simulink model "path_following_PID_v2"  (R2021b)
settings: Solver=VariableStepAuto  StartTime=0.0  StopTime=4000  RelTol=1e-3
model workspace (MAT data in the model file):
  index = 1
values from neighbouring files (symbols this model uses):
  ref = [x_ref, -y_ref]    [reference.m]
libraries: slpidlib x2
settings Model: Creator=andreagottardini  LastModifiedBy=Utente
settings DataIOCC: ReturnWorkspaceOutputs=off
settings DebuggingCC: UnconnectedInputMsg=none  UnconnectedOutputMsg=none  UnconnectedLineMsg=none
settings RTWCC: DLArmComputeVersion=20.02.1

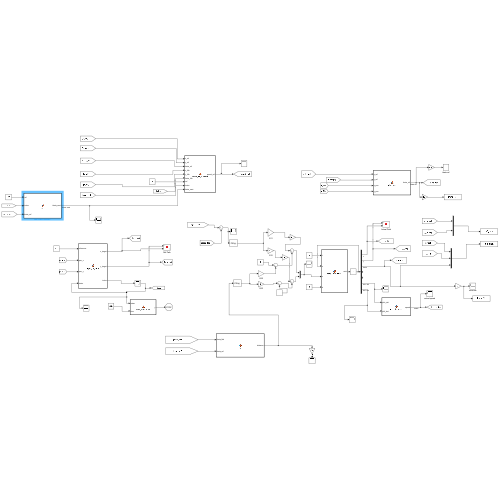
[thumbnail: Simulink's stored preview of the top-level diagram]
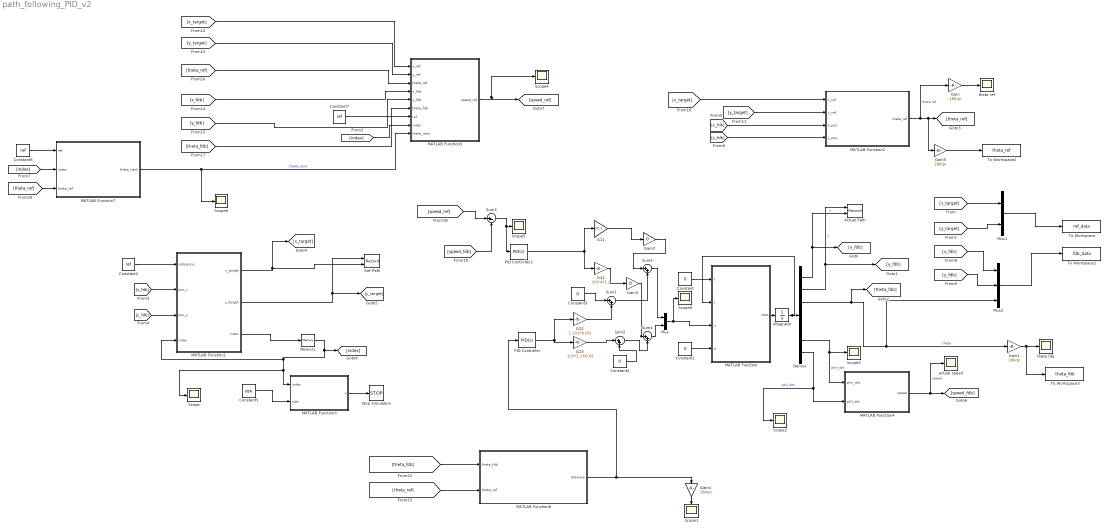
== system path_following_PID_v2 ==
  Actual Path : Record  FileSettingsInternal="{\"entries\":[{\"content\":{\"excelSettings\":{\"content\":{},\"type\":\"Streamout.ExcelSettings\"}},\"type\":\"Streamout.FileSettingStorage\",\"uuid\":\"8efc1e73-26fd-4d14-85a3-82b8725d3209\"}],\"packageUris\":[\"http://schema.mathworks.com/mf0/streamout_blocks/R2020a\"],\"version\":\"1.0\"}"  Layout=[1 1]  SignalsInternal="{\"entries\":[{\"content\":{\"signals\":[{\"content\":{\"blockPath\":[\"path_following_PID_v2/Actual Path\"],\"channel\":[],\"dimensions\":[1],\"domain\":\"path_following_PID_v2/Actual Path\",\"lineColor\":\"#ff6929\",\"plots\":[],\"port\":1,\"sid\":[\"\"],\"signalID\":63,\"signalName\":\"y\"},\"type\":\"RecordBlkView.Signal\",\"uuid\":\"c6209dd6-1482-4780-aa99-2b04ce97250a\"},{\"content\":{\"blockPath\":[\"path_following_PID_v2/Actual Path\"],\"channel\":[],\"dimensions\":[1],\"domain\":\"path_following_PID_v2/Actual Path\",\"lineColor\":\"#b746ff\",\"plots\":[],\"port\":2,\"sid\":[\"\"],\"signalID\":67,\"signalName\":\"x\"},\"type\":\"RecordBlkView.Signal\",\"uuid\":\"5d04c5e3-b3b5-4d9f-9fb0-0dadaa101284\"}]},\"type\":\"RecordBlkView.InputSignals\",\"uuid\":\"b79b6225-c0e7-4157-97cf-f8186f5de62f\"}],\"packageUris\":[\"http://schema.mathworks.com/mf0/streamout_blocks/R2020a\"],\"version\":\"1.0\"}"  VisualizationBindings="{\"xyplotplugin\":{\"info\":[{\"series\":[],\"subplotID\":1}]}}"  CompatibilityTag=XY
  Constant{,1,3..4} (4 alike) : Constant  Value=0
  Constant2 : Constant  Value=ref
  Constant5 : Constant  Value=size
  Constant6 : Constant  Value=ref
  Constant7 : Constant  Value=ref
  Demux : Demux  Outputs=7
  G11 : Gain  Gain=2*1.2
  G12 : Gain  Gain=3/2*4*1.2
  G22 : Gain  Gain=1.2/(2*0.05)
  G23 : Gain  Gain=-1/2*(1.2)/0.05
  Gain{,1,4..5} (4 alike) : Gain  Gain=180/pi
  Gain2 : Gain  Gain=0
  Gain3 : Gain  Gain=0
  Integrator : Integrator  InitialCondition=[0;0;0;0;0;0;0]
  MATLAB Function : MATLAB Function  TreatAsAtomicUnit=on
  MATLAB Function1 : MATLAB Function  TreatAsAtomicUnit=on
  MATLAB Function2 : MATLAB Function  TreatAsAtomicUnit=on
  MATLAB Function3 : MATLAB Function  TreatAsAtomicUnit=on
  MATLAB Function4 : MATLAB Function  TreatAsAtomicUnit=on
  MATLAB Function5 : MATLAB Function  TreatAsAtomicUnit=on
  MATLAB Function6 : MATLAB Function  TreatAsAtomicUnit=on
  MATLAB Function7 : MATLAB Function  TreatAsAtomicUnit=on
  Memory : Memory  InitialCondition=1
  Mux : Mux  Inputs=2
  Mux1 : Mux  Inputs=2
  Mux2 : Mux  Inputs=3
  PID Controller : slpidlib/PID Controller  Controller=PID  Form=Parallel  TimeDomain=Continuous-time  UseExternalTs=off  SampleTime=-1  IntegratorMethod=Forward Euler  FilterMethod=Forward Euler  ControllerParametersSource=internal  P=0.154648125989768  I=0.0265164152640643  D=0.207345153563612  UseFilter=on  N=572.770791824146  TunerSelectOption=Frequency Response Based  InitialConditionSource=internal  InitialConditionForIntegrator=0  InitialConditionForFilter=0  DifferentiatorICPrevScaledInput=0  ExternalReset=none  TrackingMode=off  Kt=1  LimitOutput=off  SatLimitsSource=internal  UpperSaturationLimit=inf  LowerSaturationLimit=-inf  LinearizeAsGain=on  AntiWindupMode=none  Kb=1  POutMin=[]  POutMax=[]  IOutMin=[]  IOutMax=[]  DOutMin=[]  DOutMax=[]  NOutMin=[]  NOutMax=[]  SumOutMin=[]  SumOutMax=[]  SaturationOutMin=[]  SaturationOutMax=[]  PParamMin=[]  PParamMax=[]  IParamMin=[]  IParamMax=[]  DParamMin=[]  DParamMax=[]  NParamMin=[]  NParamMax=[]  KbParamMin=[]  KbParamMax=[]  KtParamMin=[]  KtParamMax=[]  KbOutMin=[]  KbOutMax=[]  KtOutMin=[]  KtOutMax=[]  IntegratorOutMin=[]  IntegratorOutMax=[]  FilterOutMin=[]  FilterOutMax=[]  SumI1OutMin=[]  SumI1OutMax=[]  SumI2OutMin=[]  SumI2OutMax=[]  SumI3OutMin=[]  SumI3OutMax=[]  SumI4OutMin=[]  SumI4OutMax=[]  SumDOutMin=[]  SumDOutMax=[]  DifferentiatorOutMin=[]  DifferentiatorOutMax=[]  FilterDiffOutCoefMin=[]  FilterDiffOutCoefMax=[]  ReciprocalOutMin=[]  ReciprocalOutMax=[]  SumDenOutMin=[]  SumDenOutMax=[]  SumNumOutMin=[]  SumNumOutMax=[]  DivideOutMin=[]  DivideOutMax=[]  UdiffTsProdOutMin=[]  UdiffTsProdOutMax=[]  NTsProdOutMin=[]  NTsProdOutMax=[]  UintegralTsProdOutMin=[]  UintegralTsProdOutMax=[]  UngainTsProdOutMin=[]  UngainTsProdOutMax=[]  IntegratorContinuousStateAttributes=''  IntegratorStateMustResolveToSignalObject=off  IntegratorRTWStateStorageClass=Auto  FilterContinuousStateAttributes=''  FilterStateMustResolveToSignalObject=off  FilterRTWStateStorageClass=Auto  ParallelPVariant=InternalParameters  IdealPVariant=Disabled  IVariant=InternalParameters  DVariant=InternalParameters  IntegratorVariant=Continuous  SatVariant=Disabled  AWVariant=Passthrough  PCopyVariant=Disabled  TRVariant=Disabled  FdbkBlocksVariant=Forward  IdealPFdbkVariant=Disabled  SatFdbkVariant=Disabled  DerivativeFilterVariant=ContFilter  NVariant=InternalParameters  NCopyVariant=Disabled  FilterICVariant=InternalICsFilter  IntegratorICVariant=InternalICs  ExternalResetVariant=Disabled  TRSumVariant=Passthrough  SumFdbkVariant=Disabled  SumVariant=Sum_PID  TsampFilterVariant=InternalTs  TsampNgainVariant=Passthrough  TsampIntegralVariant=Passthrough  ExternalSaturationOutDataTypeStr=Inherit: Same as second input
  PID Controller1 : slpidlib/PID Controller  Controller=PID  Form=Parallel  TimeDomain=Continuous-time  UseExternalTs=off  SampleTime=-1  IntegratorMethod=Forward Euler  FilterMethod=Forward Euler  ControllerParametersSource=internal  P=0.5  I=0.01  D=0.5  UseFilter=on  N=100  TunerSelectOption=Frequency Response Based  InitialConditionSource=internal  InitialConditionForIntegrator=0  InitialConditionForFilter=0  DifferentiatorICPrevScaledInput=0  ExternalReset=none  TrackingMode=off  Kt=1  LimitOutput=off  SatLimitsSource=internal  UpperSaturationLimit=inf  LowerSaturationLimit=-inf  LinearizeAsGain=on  AntiWindupMode=none  Kb=1  POutMin=[]  POutMax=[]  IOutMin=[]  IOutMax=[]  DOutMin=[]  DOutMax=[]  NOutMin=[]  NOutMax=[]  SumOutMin=[]  SumOutMax=[]  SaturationOutMin=[]  SaturationOutMax=[]  PParamMin=[]  PParamMax=[]  IParamMin=[]  IParamMax=[]  DParamMin=[]  DParamMax=[]  NParamMin=[]  NParamMax=[]  KbParamMin=[]  KbParamMax=[]  KtParamMin=[]  KtParamMax=[]  KbOutMin=[]  KbOutMax=[]  KtOutMin=[]  KtOutMax=[]  IntegratorOutMin=[]  IntegratorOutMax=[]  FilterOutMin=[]  FilterOutMax=[]  SumI1OutMin=[]  SumI1OutMax=[]  SumI2OutMin=[]  SumI2OutMax=[]  SumI3OutMin=[]  SumI3OutMax=[]  SumI4OutMin=[]  SumI4OutMax=[]  SumDOutMin=[]  SumDOutMax=[]  DifferentiatorOutMin=[]  DifferentiatorOutMax=[]  FilterDiffOutCoefMin=[]  FilterDiffOutCoefMax=[]  ReciprocalOutMin=[]  ReciprocalOutMax=[]  SumDenOutMin=[]  SumDenOutMax=[]  SumNumOutMin=[]  SumNumOutMax=[]  DivideOutMin=[]  DivideOutMax=[]  UdiffTsProdOutMin=[]  UdiffTsProdOutMax=[]  NTsProdOutMin=[]  NTsProdOutMax=[]  UintegralTsProdOutMin=[]  UintegralTsProdOutMax=[]  UngainTsProdOutMin=[]  UngainTsProdOutMax=[]  IntegratorContinuousStateAttributes=''  IntegratorStateMustResolveToSignalObject=off  IntegratorRTWStateStorageClass=Auto  FilterContinuousStateAttributes=''  FilterStateMustResolveToSignalObject=off  FilterRTWStateStorageClass=Auto  ParallelPVariant=InternalParameters  IdealPVariant=Disabled  IVariant=InternalParameters  DVariant=InternalParameters  IntegratorVariant=Continuous  SatVariant=Disabled  AWVariant=Passthrough  PCopyVariant=Disabled  TRVariant=Disabled  FdbkBlocksVariant=Forward  IdealPFdbkVariant=Disabled  SatFdbkVariant=Disabled  DerivativeFilterVariant=ContFilter  NVariant=InternalParameters  NCopyVariant=Disabled  FilterICVariant=InternalICsFilter  IntegratorICVariant=InternalICs  ExternalResetVariant=Disabled  TRSumVariant=Passthrough  SumFdbkVariant=Disabled  SumVariant=Sum_PID  TsampFilterVariant=InternalTs  TsampNgainVariant=Passthrough  TsampIntegralVariant=Passthrough  ExternalSaturationOutDataTypeStr=Inherit: Same as second input
  Ref Path : Record  FileSettingsInternal="{\"entries\":[{\"content\":{\"excelSettings\":{\"content\":{},\"type\":\"Streamout.ExcelSettings\"}},\"type\":\"Streamout.FileSettingStorage\",\"uuid\":\"41089fd7-de7c-4e54-9a34-cb09a517867c\"}],\"packageUris\":[\"http://schema.mathworks.com/mf0/streamout_blocks/R2020a\"],\"version\":\"1.0\"}"  Layout=[1 1]  SignalsInternal="{\"entries\":[{\"content\":{\"signals\":[{\"content\":{\"blockPath\":[\"path_following_PID_v2/Ref Path\"],\"channel\":[],\"dimensions\":[1],\"domain\":\"path_following_PID_v2/Ref Path\",\"lineColor\":\"#64d413\",\"plots\":[],\"port\":1,\"sid\":[\"\"],\"signalID\":71,\"signalName\":\"MATLAB Function1:2\"},\"type\":\"RecordBlkView.Signal\",\"uuid\":\"e4a04d2a-34d2-407d-ad96-dcd9bf666eba\"},{\"content\":{\"blockPath\":[\"path_following_PID_v2/Ref Path\"],\"channel\":[],\"dimensions\":[1],\"domain\":\"path_following_PID_v2/Ref Path\",\"lineColor\":\"#ff13a6\",\"plots\":[],\"port\":2,\"sid\":[\"\"],\"signalID\":75,\"signalName\":\"MATLAB Function1:1\"},\"type\":\"RecordBlkView.Signal\",\"uuid\":\"290c8e0f-e7e2-4bad-bcf1-82738d60235b\"}]},\"type\":\"RecordBlkView.InputSignals\",\"uuid\":\"66d24341-99bc-4bed-aa77-b0ae85dd6ff0\"}],\"packageUris\":[\"http://schema.mathworks.com/mf0/streamout_blocks/R2020a\"],\"version\":\"1.0\"}"  VisualizationBindings="{\"xyplotplugin\":{\"info\":[{\"series\":[],\"subplotID\":1}]}}"  CompatibilityTag=XY
  Scope{,1..6,8} (8 alike) : Scope
  Stop Simulation : Stop
  Sum{1..2,4..5} (4 alike) : Sum  Inputs=|++
  Sum3 : Sum  Inputs=|+-
  To Workspace : ToWorkspace  VariableName=ref_data  SampleTime=-1
      settings: Save2DSignal=2-D array (concatenate along first dimension)
  To Workspace1 : ToWorkspace  VariableName=fdb_data  SampleTime=-1
      settings: Save2DSignal=2-D array (concatenate along first dimension)
  To Workspace2 : ToWorkspace  VariableName=theta_ref  SaveFormat=Timeseries  SampleTime=-1
  To Workspace3 : ToWorkspace  VariableName=theta_fdb  SaveFormat=Timeseries  SampleTime=-1
  actual speed : Scope
  theta fdb : Scope
  theta ref : Scope
  wires:
  Constant/1 -> MATLAB Function/1(t)
  Constant1/1 -> MATLAB Function/4(d)
  Integrator/1 -> MATLAB Function/2(z), Demux/1
  MATLAB Function/1(zdot) -> Integrator/1
  PID Controller/1 -> G22/1, G23/1
  Demux/1 -> Actual Path/2, [x_fdb]  "x"
  Demux/2 -> Actual Path/1, [y_fdb]  "y"
  Demux/3 -> Mux2/3, Gain1/1, [theta_fdb]  "theta"
  MATLAB Function1/1(x_target) -> [x_target], Ref Path/2
  Constant2/1 -> MATLAB Function1/1(reference)
  [x_fdb] -> MATLAB Function1/2(pos_x)
  [y_fdb] -> MATLAB Function1/3(pos_y)
  [x_fdb] -> MATLAB Function2/3(x_pos)
  [y_fdb] -> MATLAB Function2/4(y_pos)
  MATLAB Function2/1(theta_ref) -> Gain/1, Gain5/1, [theta_ref]  "theta ref"
  MATLAB Function1/2(y_target) -> Ref Path/1, [y_target]
  [x_target] -> MATLAB Function2/1(x_ref)
  [y_target] -> MATLAB Function2/2(y_ref)
  Memory/1 -> [index], Scope/1, MATLAB Function3/1(index), MATLAB Function1/4("index ")
  MATLAB Function1/3(index) -> Memory/1
  Constant5/1 -> MATLAB Function3/2(size)
  MATLAB Function3/1(y) -> Stop Simulation/1
  Sum1/1 -> Sum5/2
  Sum2/1 -> Sum4/2
  G22/1 -> Sum1/2
  G23/1 -> Sum2/1
  Constant3/1 -> Sum1/1
  Constant4/1 -> Sum2/2
  [y_fdb] -> Mux2/2
  [x_fdb] -> Mux2/1
  [y_target] -> Mux1/2
  [x_target] -> Mux1/1
  Mux1/1 -> To Workspace/1
  Mux2/1 -> To Workspace1/1
  Demux/6 -> MATLAB Function4/1(phir_dot), Scope3/1  "phir_dot"
  Demux/7 -> Scope2/1, MATLAB Function4/2(phil_dot)  "phil_dot"
  MATLAB Function4/1(speed) -> actual speed/1, [speed_fdb]  "speed"
  [x_target] -> MATLAB Function5/1(x_ref)
  [y_target] -> MATLAB Function5/2(y_ref)
  [x_fdb] -> MATLAB Function5/4(x_fdb)
  [speed_ref] -> Sum3/1
  [speed_fdb] -> Sum3/2
  Sum3/1 -> Scope5/1, PID Controller1/1
  Mux/1 -> Scope8/1, MATLAB Function/3(u)
  Sum4/1 -> Mux/2
  Sum5/1 -> Mux/1
  PID Controller1/1 -> G11/1, G12/1
  Gain/1 -> theta ref/1
  Gain1/1 -> To Workspace3/1, theta fdb/1
  [theta_fdb] -> MATLAB Function6/1(theta_fdb)
  [theta_ref] -> MATLAB Function6/2(theta_ref)
  MATLAB Function6/1(distance) -> PID Controller/1, Gain4/1
  G11/1 -> Gain2/1
  Gain2/1 -> Sum5/1
  G12/1 -> Gain3/1
  Gain3/1 -> Sum4/1
  Gain4/1 -> Scope1/1
  Gain5/1 -> To Workspace2/1
  Constant7/1 -> MATLAB Function5/7(ref)
  [index] -> MATLAB Function5/8(index)
  MATLAB Function7/1(theta_next) -> Scope6/1, MATLAB Function5/9(theta_next)  "theta_next"
  MATLAB Function5/1(speed_ref) -> Scope4/1, [speed_ref]
  [index] -> MATLAB Function7/2(index)
  Constant6/1 -> MATLAB Function7/1(ref)
  [theta_ref] -> MATLAB Function5/3(theta_ref)
  [y_fdb] -> MATLAB Function5/5(y_fdb)
  [theta_fdb] -> MATLAB Function5/6(theta_fdb)
  [theta_ref] -> MATLAB Function7/3(theta_ref)

== matlab function path_following_PID_v2/MATLAB Function1 ==
  data: reference input; x_target output; pos_x input; pos_y input; y_target output; index input; index output
function [x_target, y_target, index] = target_to_follow(reference, pos_x, pos_y,index)

current_target_x = reference(index,1);
current_target_y = reference(index,2);

distance = sqrt((current_target_x - pos_x)^2+(current_target_y - pos_y)^2);

if distance <= 0.5
    index= index + 1;
else
    index = index;
end


x_target = reference(index,1);
y_target = reference(index,2);


end

== matlab function path_following_PID_v2/MATLAB Function ==
  data: t input; z input; u input; zdot output; d input
function zdot=robot_dyn_model(t,z,u,d)

%% Read parameters, states and inputs

% Parameters
% Ic      =       th(1,1);     %
% Iw      =       th(2,1);     % 
% d       =       th(3,1);     % 
% mw      =       th(4,1);     % 
% mc      =       th(5,1);     % 
% Im      =       th(6,1);     % 
% R       =       th(7,1);     % 
% L       =       th(8,1);     % 

 Ic      =       1;     %
 Iw      =       0.1;     % 
 d       =       0.05;     % 
 mw      =       0.1;     % 
 mc      =       1;     % 
 Im      =       0.1;     % 
 R       =       0.025;     % 
 L       =       0.05;

mT = mc+2*mw;
I = Ic+mc*d^2+2*mw*L^2+2*Im;


% States
xa                  =       z(1,1);    % inertial X position (m)
ya                  =       z(2,1);    % inertial Y position (m)
theta               =       z(3,1);    % body orientation - yaw angle(rad)
phir                =       z(4,1);    % angular displacement right wheel (rad)
phil                =       z(5,1);    % angular displacement left wheel (rad)
phir_dot            =       z(6,1);    % angular velocity right wheel (rad/s)    
phil_dot            =       z(7,1);    % angular velocity left wheel (rad/s)



% Additional paramaeters
cth = cos(theta);
sth = sin(theta);

lam = [-sth     cth     0;
        cth     sth     L;
        cth     sth     -L];

b = inv(lam)*[0; R*phir_dot; R*phil_dot];

xa_dot      =    b(1,1);
ya_dot      =    b(2,1);
theta_dot   =    b(3,1);




% Inputs
taur      =       u(1,1);     % driving/braking torque right wheel (N*m)
taul      =       u(2,1);     % driving/braking torque left wheel (N*m)


%% Matrices


S = [R/(2*L)*(L*cth-d*sth) R/(2*L)*(L*cth+d*sth);
     R/(2*L)*(L*sth+d*cth) R/(2*L)*(L*sth-d*cth);
     R/(2*L)               -R/(2*L)             ;
     1                      0                   ;
     0                      1];


M_bar = [Iw+R^2/(4*L^2)*(mT*L^2+I)          R^2/(4*L^2)*(mT*L^2-I); 
        R^2/(4*L^2)*(mT*L^2-I)              Iw+R^2/(4*L^2)*(mT*L^2+I)];

V_bar = [0                              R^2/(2*L)*mc*d*theta_dot;
        -R^2/(2*L)*mc*d*theta_dot               0];



% Model equations

zdot = zeros(7,1);

zdot = [S*z(6:7,1); zeros(2,1)] + [zeros(5,2); eye(2)]*inv(M_bar)*(u-V_bar*z(6:7,1));

== matlab function path_following_PID_v2/MATLAB Function2 ==
  data: x_ref input; theta_ref output; y_ref input; x_pos input; y_pos input
function theta_ref = direction (x_ref, y_ref, x_pos, y_pos)

if (x_pos >= x_ref && abs(y_pos-y_ref)<=10^-3)
    theta_ref = pi;
elseif (abs(x_pos-x_ref)<=10^-3 && y_pos <= y_ref )
    theta_ref = pi/2;
elseif (x_pos < x_ref && abs(y_pos-y_ref)<=10^-3)
    theta_ref = 0;
elseif (abs(x_pos-x_ref)<=10^-3 && y_pos > y_ref )
    theta_ref = 3*pi/2;
elseif (x_pos<x_ref && y_pos<y_ref)
    theta_ref = atan((y_ref-y_pos)/(x_ref-x_pos));
elseif (x_pos>x_ref && y_pos<y_ref)
    theta_ref = pi-atan((y_ref-y_pos)/(x_pos-x_ref));
elseif (x_pos>x_ref && y_pos>y_ref)
    theta_ref = pi+atan((y_pos-y_ref)/(x_pos-x_ref));
else %(x_pos<x_ref && y_pos>y_ref)
    theta_ref = 2*pi-atan((y_pos-y_ref)/(x_ref-x_pos));
end

== matlab function path_following_PID_v2/MATLAB Function3 ==
  data: index input; y output; size input
function y = stop_simulation(index, size)

if (index == size)
    y = 1;
else 
    y=0;

end

== matlab function path_following_PID_v2/MATLAB Function4 ==
  data: phir_dot input; speed output; phil_dot input
function speed = compute_speed(phir_dot, phil_dot)

speed = ((phir_dot*0.025)+(phil_dot*0.025))/2;

== matlab function path_following_PID_v2/MATLAB Function5 ==
  data: x_ref input; speed_ref output; y_ref input; theta_ref input; x_fdb input; y_fdb input; theta_fdb input; ref input; index input; theta_next input
function speed_ref = speed_ref_function(x_ref, y_ref, theta_ref, x_fdb, y_fdb, theta_fdb, ref, index, theta_next)

x_next = ref(index+1,1);
y_next = ref(index+1,2);

distance_curr = sqrt((x_ref-x_fdb)^2+(y_ref-y_fdb)^2);
distance_next = sqrt((x_next-x_fdb)^2+(y_next-y_fdb)^2);

diff_curr = rem(theta_ref-theta_fdb, 2*pi);
diff_next = rem(theta_next-theta_ref, 2*pi);

if (abs(diff_curr)<=0.05)
    if (abs(diff_next)<=0.05)
        speed_ref = 0.2*distance_next;
    else
        speed_ref = 0.2*distance_curr;
    end
else
    speed_ref = 0;
end

== matlab function path_following_PID_v2/MATLAB Function6 ==
  data: theta_fdb input; theta_ref input; distance output
function distance = fcn(theta_fdb,theta_ref)

distance = rem((theta_ref - theta_fdb),2*pi);
if (distance < -pi)
    distance = (distance + 2*pi);
elseif (distance > pi)
    distance = (distance - 2*pi);

end

== matlab function path_following_PID_v2/MATLAB Function7 ==
  data: ref input; theta_next output; index input; theta_ref input
function theta_next = direction (ref, index, theta_ref)

if index < length(ref)
    x_pos = ref(index,1);
    y_pos = ref(index,2);
    
    x_ref = ref(index+1,1);
    y_ref = ref(index+1,2);
    
    if (x_pos >= x_ref && abs(y_pos-y_ref)<=10^-3)
        theta_next = pi;
    elseif (abs(x_pos-x_ref)<=10^-3 && y_pos <= y_ref )
        theta_next = pi/2;
    elseif (x_pos < x_ref && abs(y_pos-y_ref)<=10^-3)
        theta_next = 0;
    elseif (abs(x_pos-x_ref)<=10^-3 && y_pos > y_ref )
        theta_next = 3*pi/2;
    elseif (x_pos<x_ref && y_pos<y_ref)
        theta_next = atan((y_ref-y_pos)/(x_ref-x_pos));
    elseif (x_pos>x_ref && y_pos<y_ref)
        theta_next = pi-atan((y_ref-y_pos)/(x_pos-x_ref));
    elseif (x_pos>x_ref && y_pos>y_ref)
        theta_next = pi+atan((y_pos-y_ref)/(x_pos-x_ref));
    else %(x_pos<x_ref && y_pos>y_ref)
        theta_next = 2*pi-atan((y_pos-y_ref)/(x_ref-x_pos));
    end
else
    theta_next = theta_ref;
end
